simulink model "Problem_1_mod_5_counter"  (R2020b)
settings: Solver=VariableStepAuto  StartTime=0.0  StopTime=10.0  RelTol=1e-3
settings Model: Creator=baner  LastModifiedBy=baner

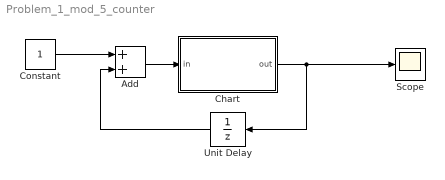
== system Problem_1_mod_5_counter ==
  Add : Sum
  Chart : Stateflow chart  TreatAsAtomicUnit=on
  Constant : Constant
  Scope : Scope
  Unit Delay : UnitDelay  SampleTime=-1  HasFrameUpgradeWarning=on
  wires:
  Chart/1(out) -> Unit Delay/1, Scope/1
  Add/1 -> Chart/1(in)
  Unit Delay/1 -> Add/2
  Constant/1 -> Add/1

== stateflow chart Problem_1_mod_5_counter/Chart ==
  (default) -> (junction 3)
  (junction 3) -> (junction 5) [order 1] : [in<=5]
  (junction 5) -> (junction 9) : {out=in;}
  (junction 9) -> (junction 11)
  (junction 3) -> (junction 7) [order 2] : [in>5]
  (junction 7) -> (junction 11) : {out=0;}
  data: in input; out output
